simulink model "UR3Simulation"  (R2016b)
settings: Solver=VariableStepAuto  StartTime=0.0  StopTime=100  RelTol=1e-3
undefined symbols (not defined in the file or in its folder): ForwardKinematics, H, InverseDynamics, Robotdynamics
settings Model: Creator=deela  LastModifiedBy=deela
settings DataIOCC: SaveFormat=Array

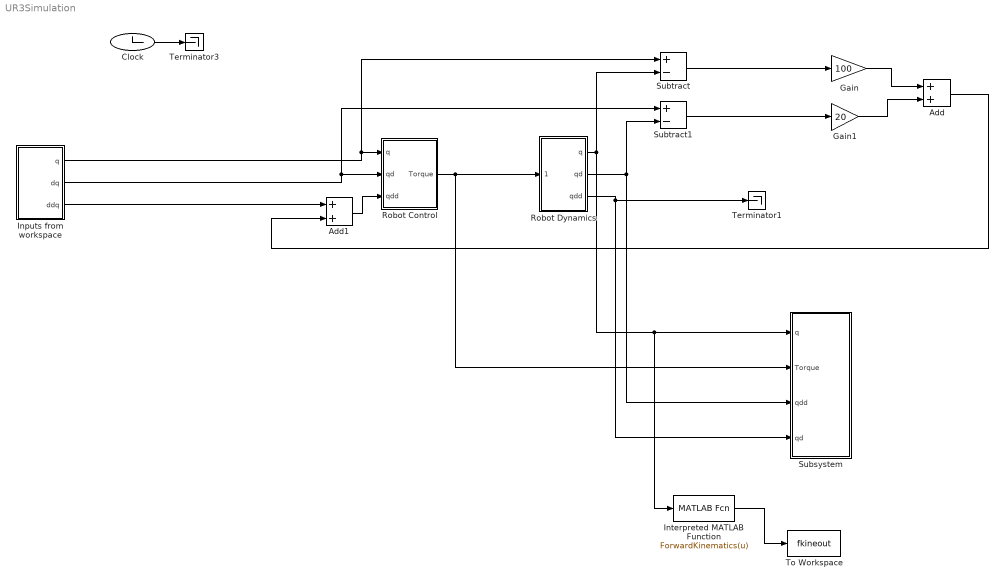
== system UR3Simulation ==
  Add : Sum
  Add1 : Sum
  Clock : Clock
  Gain : Gain  Gain=100
  Gain1 : Gain  Gain=20
  Inputs from workspace : Subsystem
  Interpreted MATLAB Function : MATLABFcn  MATLABFcn=ForwardKinematics(u)  OutputDimensions=3
  Robot Control : Subsystem
  Robot Dynamics : Subsystem
  Subsystem : Subsystem
  Subtract : Sum  Inputs=+-
  Subtract1 : Sum  Inputs=+-
  Terminator1 : Terminator
  Terminator3 : Terminator
  To Workspace : ToWorkspace  VariableName=fkineout  SaveFormat=Timeseries  SampleTime=-1
  wires:
  Inputs from workspace/1(q) -> Subtract/1, Robot Control/1(q)
  Inputs from workspace/2(dq) -> Subtract1/1, Robot Control/2(qd)
  Robot Control/1(Torque) -> Subsystem/2(Torque), Robot Dynamics/1(Torque)
  Robot Dynamics/1(q) -> Interpreted MATLAB Function/1, Subsystem/1(q), Subtract/2
  Subtract/1 -> Gain/1
  Robot Dynamics/2(qd) -> Subsystem/3(qdd), Subtract1/2
  Subtract1/1 -> Gain1/1
  Gain1/1 -> Add/2
  Gain/1 -> Add/1
  Add/1 -> Add1/2
  Add1/1 -> Robot Control/3(qdd)
  Inputs from workspace/3(ddq) -> Add1/1
  Robot Dynamics/3(qdd) -> Subsystem/4(qd), Terminator1/1
  Clock/1 -> Terminator3/1
  Interpreted MATLAB Function/1 -> To Workspace/1

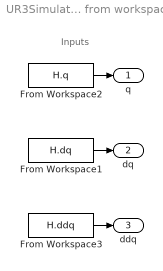
== system UR3Simulation/Inputs from workspace ==
  note: Inputs
  From Workspace1 : FromWorkspace  VariableName=H.dq  SampleTime=0.1
  From Workspace2 : FromWorkspace  VariableName=H.q  SampleTime=0.1
  From Workspace3 : FromWorkspace  VariableName=H.ddq  SampleTime=0.1
  q : Outport
  dq : Outport  Port=2
  ddq : Outport  Port=3
  wires:
  From Workspace1/1 -> dq/1
  From Workspace3/1 -> ddq/1
  From Workspace2/1 -> q/1

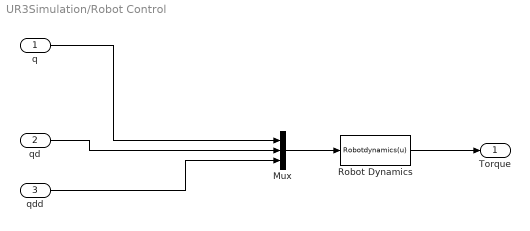
== system UR3Simulation/Robot Control ==
  q : Inport
  qd : Inport  Port=2
  qdd : Inport  Port=3
  Mux : Mux  Inputs=3
  Robot Dynamics : MATLABFcn  MATLABFcn=Robotdynamics(u)  OutputDimensions=6
  Torque : Outport
  wires:
  qd/1 -> Mux/2
  Robot Dynamics/1 -> Torque/1
  q/1 -> Mux/1
  qdd/1 -> Mux/3
  Mux/1 -> Robot Dynamics/1

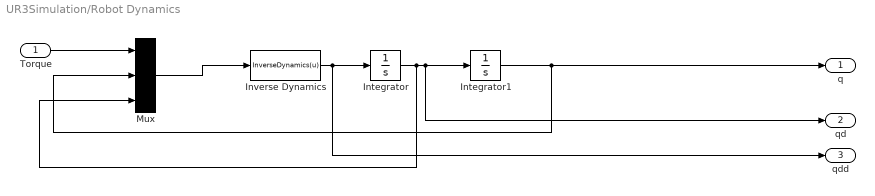
== system UR3Simulation/Robot Dynamics ==
  Torque : Inport
  Integrator : Integrator  InitialCondition=H.dq(1,2:7)
  Integrator1 : Integrator  InitialCondition=[1, 2, 3, 4, 5, 6]
  Inverse Dynamics : MATLABFcn  MATLABFcn=InverseDynamics(u)  OutputDimensions=6
  Mux : Mux  Inputs=3
  q : Outport
  qd : Outport  Port=2
  qdd : Outport  Port=3
  wires:
  Integrator1/1 -> Mux/2, q/1
  Integrator/1 -> Mux/3, qd/1, Integrator1/1
  Inverse Dynamics/1 -> qdd/1, Integrator/1
  Mux/1 -> Inverse Dynamics/1
  Torque/1 -> Mux/1

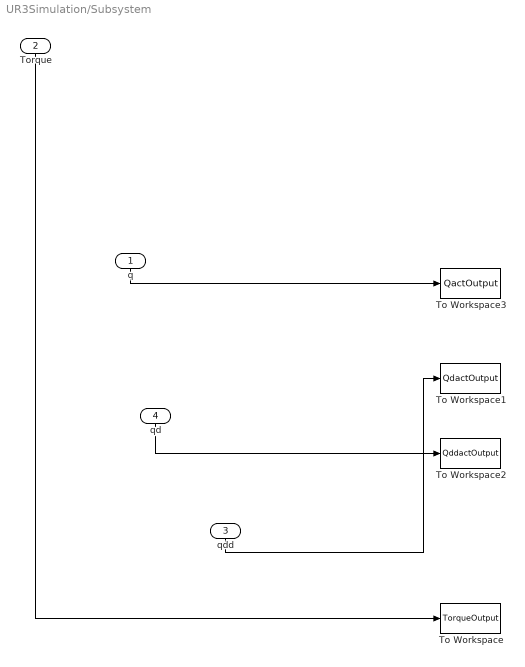
== system UR3Simulation/Subsystem ==
  q : Inport
  Torque : Inport  Port=2
  qdd : Inport  Port=3
  qd : Inport  Port=4
  To Workspace : ToWorkspace  VariableName=TorqueOutput  SaveFormat=Timeseries  SampleTime=-1
  To Workspace1 : ToWorkspace  VariableName=QdactOutput  SaveFormat=Timeseries  SampleTime=-1
  To Workspace2 : ToWorkspace  VariableName=QddactOutput  SaveFormat=Timeseries  SampleTime=-1
  To Workspace3 : ToWorkspace  VariableName=QactOutput  SaveFormat=Timeseries  SampleTime=0.1
  wires:
  Torque/1 -> To Workspace/1
  q/1 -> To Workspace3/1
  qd/1 -> To Workspace2/1
  qdd/1 -> To Workspace1/1
